simulink model "FOC_Ctrl_CodeModel"  (R2020b)
settings: Solver=FixedStepDiscrete  StartTime=0.0  StopTime=10.0  FixedStep=Tctr  RelTol=1e-3
settings Model: Creator=k  LastModifiedBy=k
settings OptimizationCC: DefaultParameterBehavior=Inlined  EnhancedBackFolding=on  PassReuseOutputArgsAs=Individual arguments  ZeroExternalMemoryAtStartup=off  ZeroInternalMemoryAtStartup=off  OptimizeBlockOrder=speed  DifferentSizesBufferReuse=on  OptimizationCustomize=off  EfficientTunableParamExpr=on
settings DebuggingCC: ParameterTunabilityLossMsg=error
settings SFSimCC: MATLABDynamicMemAlloc=off
settings RTWCC: Description=Embedded Coder  SystemTargetFile=ert.tlc  GenCodeOnly=on  TemplateMakefile=ert_default_tmf
settings CodeAppCC: ForceParamTrailComments=on  IgnoreCustomStorageClasses=off  OperatorAnnotations=on  SimulinkDataObjDesc=on  SFDataObjDesc=on  InsertBlockDesc=on
settings ERTTargetCC: TargetLangStandard=C99 (ISO)  GenerateSampleERTMain=on  InlinedParameterPlacement=NonHierarchical  ERTCustomFileTemplate=example_file_process.tlc

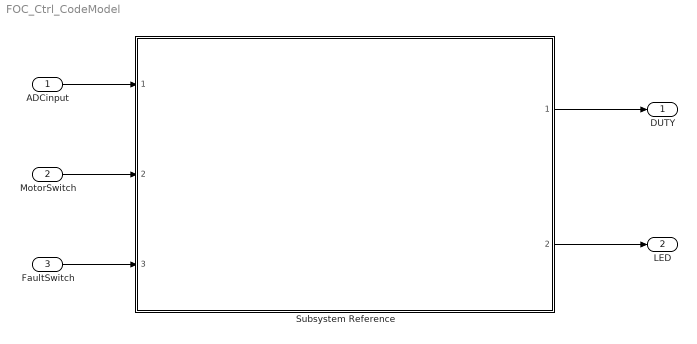
== system FOC_Ctrl_CodeModel ==
  ADCinput : Inport  OutDataTypeStr=uint16  PortDimensions=5
  MotorSwitch : Inport  Port=2  OutDataTypeStr=boolean  PortDimensions=1
  FaultSwitch : Inport  Port=3  OutDataTypeStr=boolean  PortDimensions=1
  Subsystem Reference : Subsystem  ReferencedSubsystem=FOC_Sub_StateMch
  DUTY : Outport  PortDimensions=3
  LED : Outport  Port=2  PortDimensions=3
  wires:
  FaultSwitch/1 -> Subsystem Reference/3
  MotorSwitch/1 -> Subsystem Reference/2
  ADCinput/1 -> Subsystem Reference/1
  Subsystem Reference/1 -> DUTY/1
  Subsystem Reference/2 -> LED/1
